simulink model "Model_Simulation"  (R2016a)
settings: Solver=FixedStepAuto  StartTime=0.0  StopTime=5  FixedStep=2e-6  RelTol=1e-3
values from neighbouring files (symbols this model uses):
  C = 3060e-6    (= 0.00306)    [Controle_Inversor_UR_D.m]
  Ki_i_disc = wc*Rf    (= 44.2477838534)    [Controle_Inversor_UR_D.m]
  Ki_i_disc_b = wc_b*Rb/Vdc    (= 0.0983284085631)    [Controle_Inversor_UR_D.m]
  Ki_q_disc = wq/H    [Controle_Inversor_UR_D.m]
  Ki_v_disc_b = wc_bv/Req    (= 14.5799013102)    [Controle_Inversor_UR_D.m]
  Ki_vdc_disc = ((wvdc)^2*C)/Gt    [Controle_Inversor_UR_D.m]
  Kp_i_disc = wc*Lf    (= 2.19688771906)    [Controle_Inversor_UR_D.m]
  Kp_i_disc_b = wc_b*Lb/Vdc    (= 0.00545604673435)    [Controle_Inversor_UR_D.m]
  Kp_q_disc = Ki_q_disc*(Lf/Kp_i_disc)    [Controle_Inversor_UR_D.m]
  Kp_v_disc_b = wc_bv*Cin    (= 0.0356301510224)    [Controle_Inversor_UR_D.m]
  Kp_vdc_disc = (2*ksi_vdc*wvdc*C)/Gt    [Controle_Inversor_UR_D.m]
  Lf = (0.0012+2.8949e-04)    (= 0.00148949)    [Controle_Inversor_UR_D.m]
  Tsw = 1/fsw    (= 0.0002)    [Controle_Inversor_UR_D.m]
  w = 2*pi*60    (= 376.991118431)    [Controle_Inversor_UR_D.m]
undefined symbols (not defined in the file or in its folder): D1, dEgdT, Delta, EgRef, gcbh, k1, Rsh_array5pc, sigbuilder_block, sps_rtmsupport, Tref_K, VT_ref
libraries: powerlib x179, simulink x14, powerlib_meascontrol x13, spsPVarrayModel x12
(part 6 of 20)

== system Model_Simulation/Subsystem2/ABC2DQ ==
  ABC. : Inport
  Fase : Inport  Port=2
  Demux1 : Demux  Outputs=3
  Fcn1 : Fcn  Commented=on  Expr=sin(u[1])*u(2)+sin(u[1]-(2*pi/3))*u(3)+sin(u[1]+(2*pi/3))*u(4)
  Fcn2 : Fcn  Commented=on  Expr=cos(u[1])*u(2)+cos(u[1]-(2*pi/3))*u(3)+cos(u[1]+(2*pi/3))*u(4);
  Gain : Gain  Commented=on  Gain=2/3
  Gain4 : Gain  Commented=on  Gain=2/3
  Transformada de Clarke abc para alfa_beta_zero : MATLAB Function  TreatAsAtomicUnit=on
  Transformada de Park alfa_beta_zero para dq0 : MATLAB Function  TreatAsAtomicUnit=on
  Vd : Outport
  Vq : Outport  Port=2
  wires:
  Gain4/1 -> ?
  Fcn1/1 -> Gain4/1
  Gain/1 -> ?  "Vd"
  Fcn2/1 -> Gain/1
  ABC./1 -> Demux1/1
  Demux1/2 -> Transformada de Clarke abc para alfa_beta_zero/2(fb)
  Demux1/1 -> Transformada de Clarke abc para alfa_beta_zero/1(fa)
  Demux1/3 -> Transformada de Clarke abc para alfa_beta_zero/3(fc)
  Transformada de Clarke abc para alfa_beta_zero/1(falfa) -> Transformada de Park alfa_beta_zero para dq0/1(falfa)
  Transformada de Clarke abc para alfa_beta_zero/2(fbeta) -> Transformada de Park alfa_beta_zero para dq0/2(fbeta)
  Transformada de Clarke abc para alfa_beta_zero/3(fzero) -> Transformada de Park alfa_beta_zero para dq0/3(fzero)
  Fase/1 -> Transformada de Park alfa_beta_zero para dq0/4(theta)
  Transformada de Park alfa_beta_zero para dq0/1(fd) -> Vd/1
  Transformada de Park alfa_beta_zero para dq0/2(fq) -> Vq/1

== system Model_Simulation/Subsystem2/ABC2DQ3 ==
  ABC. : Inport
  Fase : Inport  Port=2
  Demux1 : Demux  Outputs=3
  Fcn1 : Fcn  Commented=on  Expr=sin(u[1])*u(2)+sin(u[1]-(2*pi/3))*u(3)+sin(u[1]+(2*pi/3))*u(4)
  Fcn2 : Fcn  Commented=on  Expr=cos(u[1])*u(2)+cos(u[1]-(2*pi/3))*u(3)+cos(u[1]+(2*pi/3))*u(4);
  Gain : Gain  Commented=on  Gain=2/3
  Gain4 : Gain  Commented=on  Gain=2/3
  Transformada de Clarke abc para alfa_beta_zero : MATLAB Function  TreatAsAtomicUnit=on
  Transformada de Park alfa_beta_zero para dq0 : MATLAB Function  TreatAsAtomicUnit=on
  Id : Outport
  Iq : Outport  Port=2
  wires:
  Transformada de Park alfa_beta_zero para dq0/2(fq) -> Iq/1
  Transformada de Park alfa_beta_zero para dq0/1(fd) -> Id/1
  Fase/1 -> Transformada de Park alfa_beta_zero para dq0/4(theta)
  Transformada de Clarke abc para alfa_beta_zero/3(fzero) -> Transformada de Park alfa_beta_zero para dq0/3(fzero)
  Transformada de Clarke abc para alfa_beta_zero/2(fbeta) -> Transformada de Park alfa_beta_zero para dq0/2(fbeta)
  Transformada de Clarke abc para alfa_beta_zero/1(falfa) -> Transformada de Park alfa_beta_zero para dq0/1(falfa)
  Demux1/3 -> Transformada de Clarke abc para alfa_beta_zero/3(fc)
  Demux1/1 -> Transformada de Clarke abc para alfa_beta_zero/1(fa)
  Demux1/2 -> Transformada de Clarke abc para alfa_beta_zero/2(fb)
  ABC./1 -> Demux1/1
  Fcn2/1 -> Gain/1
  Gain/1 -> ?  "Vd"
  Fcn1/1 -> Gain4/1
  Gain4/1 -> ?

== system Model_Simulation/Subsystem2/Arranjo 21 strings em paralelo com 43 módulos em série Vmp = 43 x 30,6 = 1315,8 V Imp = 8,32 x 21 = 174,72 A 229.896,576 W ==
  note: Vd=V_PV + Rs*I_PV
  S : Inport
  TempC : Inport  Port=2
  Add1 : Sum
  Diode Rsh : Subsystem
      mask Display:
      | plot(-75,-50,100,150, [-15 -15 43 -15 -15 -75],[50 8 50 92 50 50], ...
      |     [43 43],[8 94],[100 43], [50 50])
  Goto Tag Visibility : GotoTagVisibility  GotoTag=S_Sref
  Goto Tag Visibility1 : GotoTagVisibility  GotoTag=Vd
  Goto Tag Visibility2 : GotoTagVisibility  GotoTag=Tcell_K
  I Filter : spsPVarrayModel/No  VariantControl=Variant1
  IL : powerlib/Electrical Sources/Controlled Current Source  Initialize=on  Source_Type=AC  Amplitude=0  Phase=0  Frequency=0  Measurements=None
  IL ctrl : Subsystem
  I_PV : powerlib/Measurements/Current Measurement  PhasorSimulation=off  OutputType=Complex  PSBequivalent=0
  Product2 : Product  Inputs=**  RndMeth=Zero
  Rs_array : powerlib/Elements/Series RLC Branch  LConnTagsString=__new0  RConnTagsString=__new0  BranchType=R  Resistance=Rs*Nser/Npar  Inductance=1e-3  SetiL0=off  InitialCurrent=0  Capacitance=1e-6  Setx0=off  InitialVoltage=0  Measurements=None
  Rs_array_ : Constant  Value=Rs*Nser/Npar
  Rsh_array For 0.05*Sref : powerlib/Elements/Series RLC Branch  LConnTagsString=__new0  RConnTagsString=__new0  BranchType=R  Resistance=Rsh_array5pc  Inductance=1e-3  SetiL0=off  InitialCurrent=0  Capacitance=1e-6  Setx0=off  InitialVoltage=0  Measurements=None
  V Filter : spsPVarrayModel/No  VariantControl=Variant1
  V_PV : powerlib/Measurements/Voltage Measurement  PhasorSimulation=off  OutputType=Complex  PSBequivalent=0
  + : PMIOPort  Port=1  Side=Right
  - : PMIOPort  Port=2  Side=Right
  tag scope: Vd=scoped
  wires:
  TempC/1 -> IL ctrl/1(Temperature)  "Temperature (deg C)"
  S/1 -> IL ctrl/2(Irradiance)  "Irradiance (W/m2)"
  Add1/1 -> [Vd]  "Vd"
  I_PV/1 -> I Filter/1  "I_PV"
  Product2/1 -> Add1/2
  Rs_array_/1 -> Product2/2
  IL ctrl/1(IL) -> IL/1
  V_PV/1 -> V Filter/1
  I Filter/1 -> Product2/1  "I_PV"
  V Filter/1 -> Add1/1  "V_PV"
  connections:
  +/RConn1 -- I_PV/RConn1 -- V_PV/LConn1
  Diode Rsh/LConn1 -- Rs_array/LConn1 -- Rsh_array For 0.05*Sref/LConn1 -- IL/RConn1
  V_PV/LConn2 -- -/RConn1 -- Rsh_array For 0.05*Sref/RConn1 -- Diode Rsh/RConn1 -- IL/LConn1
  Rs_array/RConn1 -- I_PV/LConn1

== system Model_Simulation/Subsystem2/Controlador AVR ==
  Vd : Inport
  AVR backup : Subsystem  Commented=on
  AVR modificado : Subsystem
  Clock : Clock
  Constant2 : Constant  Value=0
  Scope3 : Scope  NumInputPorts=2
  Switch3 : Switch  Threshold=0.01
  MO : Outport
  S : Outport  Port=2
  wires:
  Vd/1 -> AVR modificado/1(Vd)
  AVR modificado/1(S) -> S/1, Scope3/1
  Clock/1 -> Switch3/2
  AVR modificado/2(MO) -> Switch3/1
  Constant2/1 -> Switch3/3
  Switch3/1 -> Scope3/2, MO/1

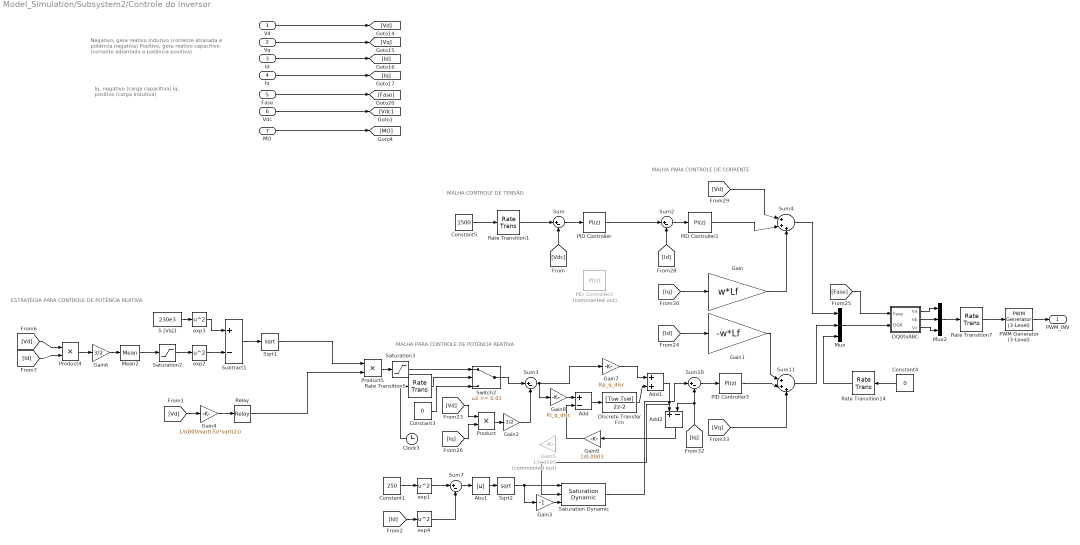
== system Model_Simulation/Subsystem2/Controle do inversor ==
  note: MALHA CONTROLE DE TENSÃO
  note: MALHA PARA CONTROLE DE CORRENTE
  note: ESTRATÉGIA PARA CONTROLE DE POTÊNCIA REATIVA
  note: Negativo, gera reativo indutivo (corrente atrasada e potência negativa)
      | Positivo, gera reativo capacitivo (corrente adiantada e potência positiva)
  note: Iq, negativo (carga capacitiva)
      | Iq, positivo (carga indutiva)
  note: MALHA PARA CONTROLE DE POTÊNCIA REATIVA
  Vd : Inport
  Vq : Inport  Port=2
  Id : Inport  Port=3
  Iq : Inport  Port=4
  Fase : Inport  Port=5
  Vdc : Inport  Port=6
  MO : Inport  Port=7
  Abs1 : Abs
  Add : Sum  Inputs=+-
  Add1 : Sum
  Add2 : Sum  Inputs=+-
  Clock3 : Clock
  Constant1 : Constant  Value=250
  Constant3 : Constant  Value=0
  Constant4 : Constant  Value=0
  Constant5 : Constant  Value=1500
  DQ0toABC : Subsystem
  Discrete Transfer Fcn : DiscreteTransferFcn  Numerator=[Tsw Tsw]  Denominator=[2 -2]
  Gain : Gain  Gain=w*Lf
  Gain1 : Gain  Gain=-w*Lf
  Gain2 : Gain  Gain=-3/2
  Gain3 : Gain  Gain=-1
  Gain4 : Gain  Gain=1/((800/sqrt(3))*sqrt(2))
  Gain5 : Gain  Commented=on  Gain=1/0.0005
  Gain6 : Gain  Gain=3/2
  Gain7 : Gain  Gain=Kp_q_disc
  Gain8 : Gain  Gain=Ki_q_disc
  Gain9 : Gain  Gain=1/0.0003
  Mean2 : powerlib_meascontrol/Measurements/Mean  Freq=10  Vinit=0  Ts=Tsw
  Mux : Mux  Inputs=3
  Mux2 : Mux  Inputs=3
  PID Controller : simulink/Continuous/PID Controller  Controller=PI  TimeDomain=Discrete-time  SampleTime=-1  IntegratorMethod=Trapezoidal  FilterMethod=Forward Euler  Form=Parallel  UseFilter=on  ControllerParametersSource=internal  P=-Kp_vdc_disc  I=-Ki_vdc_disc  D=0  N=100  InitialConditionSource=internal  InitialConditionForIntegrator=0  InitialConditionForFilter=0  ExternalReset=none  LimitOutput=off  UpperSaturationLimit=inf  LowerSaturationLimit=-inf  LinearizeAsGain=on  AntiWindupMode=none  Kb=1  TrackingMode=off  Kt=1  PParamMin=[]  PParamMax=[]  IParamMin=[]  IParamMax=[]  DParamMin=[]  DParamMax=[]  NParamMin=[]  NParamMax=[]  KbParamMin=[]  KbParamMax=[]  KtParamMin=[]  KtParamMax=[]  POutMin=[]  POutMax=[]  IOutMin=[]  IOutMax=[]  DOutMin=[]  DOutMax=[]  NOutMin=[]  NOutMax=[]  KbOutMin=[]  KbOutMax=[]  KtOutMin=[]  KtOutMax=[]  IntegratorOutMin=[]  IntegratorOutMax=[]  FilterOutMin=[]  FilterOutMax=[]  SumOutMin=[]  SumOutMax=[]  SumI1OutMin=[]  SumI1OutMax=[]  SumI2OutMin=[]  SumI2OutMax=[]  SumI3OutMin=[]  SumI3OutMax=[]  SumDOutMin=[]  SumDOutMax=[]  SaturationOutMin=[]  SaturationOutMax=[]  IntegratorContinuousStateAttributes=''  IntegratorStateMustResolveToSignalObject=off  IntegratorRTWStateStorageClass=Auto  FilterContinuousStateAttributes=''  FilterStateMustResolveToSignalObject=off  FilterRTWStateStorageClass=Auto  DifferentiatorICPrevScaledInput=0  DifferentiatorOutMin=[]  DifferentiatorOutMax=[]
  PID Controller1 : simulink/Continuous/PID Controller  Controller=PI  TimeDomain=Discrete-time  SampleTime=-1  IntegratorMethod=Trapezoidal  FilterMethod=Forward Euler  Form=Parallel  UseFilter=on  ControllerParametersSource=internal  P=Kp_i_disc  I=Ki_i_disc  D=0  N=100  InitialConditionSource=internal  InitialConditionForIntegrator=0  InitialConditionForFilter=0  ExternalReset=none  LimitOutput=off  UpperSaturationLimit=inf  LowerSaturationLimit=-inf  LinearizeAsGain=on  AntiWindupMode=none  Kb=1  TrackingMode=off  Kt=1  PParamMin=[]  PParamMax=[]  IParamMin=[]  IParamMax=[]  DParamMin=[]  DParamMax=[]  NParamMin=[]  NParamMax=[]  KbParamMin=[]  KbParamMax=[]  KtParamMin=[]  KtParamMax=[]  POutMin=[]  POutMax=[]  IOutMin=[]  IOutMax=[]  DOutMin=[]  DOutMax=[]  NOutMin=[]  NOutMax=[]  KbOutMin=[]  KbOutMax=[]  KtOutMin=[]  KtOutMax=[]  IntegratorOutMin=[]  IntegratorOutMax=[]  FilterOutMin=[]  FilterOutMax=[]  SumOutMin=[]  SumOutMax=[]  SumI1OutMin=[]  SumI1OutMax=[]  SumI2OutMin=[]  SumI2OutMax=[]  SumI3OutMin=[]  SumI3OutMax=[]  SumDOutMin=[]  SumDOutMax=[]  SaturationOutMin=[]  SaturationOutMax=[]  IntegratorContinuousStateAttributes=''  IntegratorStateMustResolveToSignalObject=off  IntegratorRTWStateStorageClass=Auto  FilterContinuousStateAttributes=''  FilterStateMustResolveToSignalObject=off  FilterRTWStateStorageClass=Auto  DifferentiatorICPrevScaledInput=0  DifferentiatorOutMin=[]  DifferentiatorOutMax=[]
  PID Controller2 : simulink/Continuous/PID Controller  Commented=on  Controller=PI  TimeDomain=Discrete-time  SampleTime=-1  IntegratorMethod=Trapezoidal  FilterMethod=Forward Euler  Form=Parallel  UseFilter=on  ControllerParametersSource=internal  P=Kp_q_disc  I=Ki_q_disc  D=0  N=100  InitialConditionSource=internal  InitialConditionForIntegrator=0  InitialConditionForFilter=0  ExternalReset=none  LimitOutput=off  UpperSaturationLimit=inf  LowerSaturationLimit=-inf  LinearizeAsGain=on  AntiWindupMode=back-calculation  Kb=1  TrackingMode=off  Kt=1  PParamMin=[]  PParamMax=[]  IParamMin=[]  IParamMax=[]  DParamMin=[]  DParamMax=[]  NParamMin=[]  NParamMax=[]  KbParamMin=[]  KbParamMax=[]  KtParamMin=[]  KtParamMax=[]  POutMin=[]  POutMax=[]  IOutMin=[]  IOutMax=[]  DOutMin=[]  DOutMax=[]  NOutMin=[]  NOutMax=[]  KbOutMin=[]  KbOutMax=[]  KtOutMin=[]  KtOutMax=[]  IntegratorOutMin=[]  IntegratorOutMax=[]  FilterOutMin=[]  FilterOutMax=[]  SumOutMin=[]  SumOutMax=[]  SumI1OutMin=[]  SumI1OutMax=[]  SumI2OutMin=[]  SumI2OutMax=[]  SumI3OutMin=[]  SumI3OutMax=[]  SumDOutMin=[]  SumDOutMax=[]  SaturationOutMin=[]  SaturationOutMax=[]  IntegratorContinuousStateAttributes=''  IntegratorStateMustResolveToSignalObject=off  IntegratorRTWStateStorageClass=Auto  FilterContinuousStateAttributes=''  FilterStateMustResolveToSignalObject=off  FilterRTWStateStorageClass=Auto  DifferentiatorICPrevScaledInput=0  DifferentiatorOutMin=[]  DifferentiatorOutMax=[]
  PID Controller3 : simulink/Continuous/PID Controller  Controller=PI  TimeDomain=Discrete-time  SampleTime=-1  IntegratorMethod=Trapezoidal  FilterMethod=Forward Euler  Form=Parallel  UseFilter=on  ControllerParametersSource=internal  P=Kp_i_disc  I=Ki_i_disc  D=0  N=100  InitialConditionSource=internal  InitialConditionForIntegrator=0  InitialConditionForFilter=0  ExternalReset=none  LimitOutput=off  UpperSaturationLimit=inf  LowerSaturationLimit=-inf  LinearizeAsGain=on  AntiWindupMode=none  Kb=1  TrackingMode=off  Kt=1  PParamMin=[]  PParamMax=[]  IParamMin=[]  IParamMax=[]  DParamMin=[]  DParamMax=[]  NParamMin=[]  NParamMax=[]  KbParamMin=[]  KbParamMax=[]  KtParamMin=[]  KtParamMax=[]  POutMin=[]  POutMax=[]  IOutMin=[]  IOutMax=[]  DOutMin=[]  DOutMax=[]  NOutMin=[]  NOutMax=[]  KbOutMin=[]  KbOutMax=[]  KtOutMin=[]  KtOutMax=[]  IntegratorOutMin=[]  IntegratorOutMax=[]  FilterOutMin=[]  FilterOutMax=[]  SumOutMin=[]  SumOutMax=[]  SumI1OutMin=[]  SumI1OutMax=[]  SumI2OutMin=[]  SumI2OutMax=[]  SumI3OutMin=[]  SumI3OutMax=[]  SumDOutMin=[]  SumDOutMax=[]  SaturationOutMin=[]  SaturationOutMax=[]  IntegratorContinuousStateAttributes=''  IntegratorStateMustResolveToSignalObject=off  IntegratorRTWStateStorageClass=Auto  FilterContinuousStateAttributes=''  FilterStateMustResolveToSignalObject=off  FilterRTWStateStorageClass=Auto  DifferentiatorICPrevScaledInput=0  DifferentiatorOutMin=[]  DifferentiatorOutMax=[]
  PWM Generator (3-Level) : powerlib_meascontrol/Pulse & Signal Generators/PWM Generator (3-Level)  ModulatorType=Three-phase bridge (12 pulses)  ModulatorMode=Unsynchronized  nF=27  Fc=5e3  ModulatingSignals=off  m=0.8  Freq=60  Phase=0  Ts=2e-6
  Product : Product
  Product4 : Product
  Product5 : Product
  Rate Transition1 : RateTransition  OutPortSampleTime=Tsw
  Rate Transition14 : RateTransition  OutPortSampleTime=Tsw
  Rate Transition5 : RateTransition  OutPortSampleTime=Tsw
  Rate Transition7 : RateTransition  OutPortSampleTime=2e-6
  Relay : Relay  OnSwitchValue=1.1  OffSwitchValue=0.1  OnOutputValue=-1  OffOutputValue=1
  S [Va]1 : Constant  Value=230e3
  Saturation Dynamic : simulink/Discontinuities/Saturation Dynamic  OutMin=[]  OutMax=[]  OutDataTypeStr=Inherit: Same as second input  OutDataType=fixdt(1, 16)  OutScaling=2^-10  DoSatur=off
  Saturation2 : Saturate  UpperLimit=230e3  LowerLimit=0
  Saturation3 : Saturate  UpperLimit=230e3  LowerLimit=-230e3
  Sqrt1 : Sqrt  SaturateOnIntegerOverflow=on
  Sqrt2 : Sqrt  SaturateOnIntegerOverflow=on
  Subtract1 : Sum  Inputs=+-
  Sum{,2..3,7,10} (5 alike) : Sum  Inputs=|+-
  Sum11 : Sum  Inputs=|+++
  Sum4 : Sum  Inputs=|+++
  Switch2 : Switch  Threshold=0.01
  exp{1..4} (4 alike) : Math  Operator=square  SaturateOnIntegerOverflow=on
  PWM_INV : Outport
  wires:
  [Iq] -> Gain/1
  Id/1 -> [Id]
  [Vd] -> Sum4/1
  Product/1 -> Gain2/1
  [Iq] -> Product/2
  Vd/1 -> [Vd]
  Iq/1 -> [Iq]
  [Id] -> Gain1/1
  Fase/1 -> [Fase]
  [Vdc] -> Sum/2
  [Vd] -> Product/1
  Vq/1 -> [Vq]
  [Id] -> Sum2/2
  [Iq] -> Add2/2, Sum10/2
  PID Controller3/1 -> Sum11/2
  [Vq] -> Sum11/3
  Sum/1 -> PID Controller/1
  Vdc/1 -> [Vdc]
  [Id] -> Product4/2
  [Vd] -> Product4/1
  Product4/1 -> Gain6/1
  Gain6/1 -> Mean2/1
  Saturation2/1 -> exp2/1
  exp2/1 -> Subtract1/2
  exp3/1 -> Subtract1/1
  S [Va]1/1 -> exp3/1
  Subtract1/1 -> Sqrt1/1
  Relay/1 -> Product5/2
  Sum2/1 -> PID Controller1/1
  [Fase] -> DQ0toABC/1(Fase)
  Gain/1 -> Sum4/3
  Constant5/1 -> Rate Transition1/1
  Constant4/1 -> Rate Transition14/1
  Mux/1 -> DQ0toABC/2(DQ0)
  Sum4/1 -> Mux/1
  Sum11/1 -> Mux/2
  Sum10/1 -> PID Controller3/1
  Mean2/1 -> Saturation2/1
  Clock3/1 -> Rate Transition5/1
  MO/1 -> [MO]
  Sqrt1/1 -> Product5/1
  Constant1/1 -> exp1/1
  exp1/1 -> Sum7/1
  exp4/1 -> Sum7/2
  [Id] -> exp4/1
  Sqrt2/1 -> Gain3/1, Saturation Dynamic/1
  Gain3/1 -> Saturation Dynamic/3
  PID Controller1/1 -> Sum4/2
  PID Controller/1 -> Sum2/1
  Mux2/1 -> Rate Transition7/1
  PWM Generator (3-Level)/1 -> PWM_INV/1
  DQ0toABC/1(Va) -> Mux2/1
  DQ0toABC/2(Vb) -> Mux2/2
  DQ0toABC/3(Vc) -> Mux2/3
  Sum7/1 -> Abs1/1
  Abs1/1 -> Sqrt2/1
  Rate Transition7/1 -> PWM Generator (3-Level)/1
  Rate Transition14/1 -> Mux/3
  Rate Transition1/1 -> Sum/1
  [Vd] -> Gain4/1
  Gain4/1 -> Relay/1
  Gain8/1 -> Add/1
  Add/1 -> Discrete Transfer Fcn/1
  Discrete Transfer Fcn/1 -> Add1/2
  Add1/1 -> Saturation Dynamic/2, Add2/1
  Add2/1 -> Gain9/1
  Gain9/1 -> Add/2
  Gain1/1 -> Sum11/1
  Constant3/1 -> Switch2/3
  Gain7/1 -> Add1/1
  Switch2/1 -> Sum3/1
  Gain2/1 -> Sum3/2
  Product5/1 -> Saturation3/1
  Rate Transition5/1 -> Switch2/2
  Sum3/1 -> Gain7/1, Gain8/1
  Saturation Dynamic/1 -> Sum10/1
  Saturation3/1 -> Switch2/1
